simulink library "dsparch4"  (Simulink 8.0)
settings: Solver=ode45  SolverMode=SingleTasking  StartTime=0.0  StopTime=10.0  RelTol=1e-3
values from neighbouring files (symbols this model uses):
  a = ver('dsp')    [aboutdspsystbx.m]    (also in dsparch3Transform.m = localGetVal(inData.InstanceData, 'den', '1'); dspddes3Transform.m = sprintf('getYuleWalkerIIRFilterDesignOutput(; dspfdes.m = []; dsprprim.m = a-Mi)
  b = tmp(end-3:end)    [aboutdspsystbx.m]    (also in dsparch3Transform.m = localGetVal(inData.InstanceData, 'num', '[1 2]'); dspcsum.m = find_system(blk,'LookUnderMasks','all', 'FollowLinks','on', ; dspddes3Transform.m = sprintf('; dspfdes.m = [])
  c = []    [dspfdes.m]    (also in hdldspblks_control.m = hdlnewcontrol(mfilename); midicontrols.m = cell(1,midiCountDevices); midiid.m = onCleanup(@()cleanup(cids)))
  d = docroot    [dspbhelp.m]    (also in dspfdes.m = []; dsprprim.m = ['x[' num2str(Mi) 'n/' num2str(Li) ']'])
  D = D + B    [rebuffer_delay.m]
  H = reshape(H,Li,Mi*Ni)    [dsprprim.m]
  L = h.Length    [maxstep.m]    (also in msepred.m; msesim.m)
  M = 1    [msepred.m]    (also in msesim.m)
  N = str2double(s)    [dspcsum.m]    (also in dspddes3Transform.m = sprintf('; dspwdes.m = varargin{2}; if isempty(N), N=64; end)
undefined symbols (not defined in the file or in its folder): bitrevorder, dspblkfdatool
undefined symbols (not defined in the file): dfilt
libraries: dspmtrx3 x7, dspxfrm3 x4, dspsigattribs x3, dspsigops x2, dsparch4 x1
settings Model: FPTRunName=Active  Creator=hshivaku  LastModifiedBy=schim  ExtModeAutoUpdateStatusClock=off

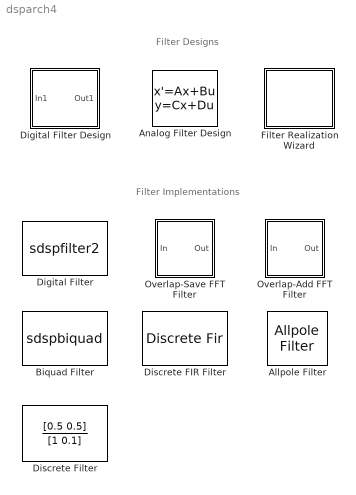
== system dsparch4 ==
  note: Filter Designs
  note: Filter Implementations
  Allpole Filter : AllpoleFilter
  Analog Filter Design : StateSpace  A=a  B=b  C=c  D=d  mask(Analog Filter Design){method=Butterworth, filttype=Lowpass, N=8, Wlo=30, Whi=80, Rp=2, Rs=40}
      mask prompts: method "Design method:"; filttype "Filter type:"; N "Filter order:"; Wlo "Passband edge frequency (rad/s):"; Whi "(unused)"; Rp "Passband ripple in dB:"; Rs "Stopband attenuation in dB:"
      mask help: Design one of several standard analog filters, implemented in state-space form.
      mask init:
      | [a,b,c,d,h,w,str]=dspblkanalog('design', method,filttype,N,Wlo,Whi,Rp,Rs);
      mask Help: eval('blocksethelp');
      mask TypeOptions method: Butterworth | Chebyshev I | Chebyshev II | Elliptic | Bessel
      mask Callback method: dspblkanalog
      mask TypeOptions filttype: Lowpass | Highpass | Bandpass | Bandstop
      mask Callback filttype: dspblkanalog
      mask Display: plot(w,h); text(.05,.9,str);
  Biquad Filter : S-Function  DialogController=dspdialog.BiquadFilter  DialogControllerArgs=DataTag1  FunctionName=sdspbiquad  Parameters=a.CoeffSource,a.FilterStruct,a.SOSCoeffs,a.ScaleValues,a.OptimizeScaleValues,a.ScaleValueMode,a.IC,a.ICnum,a.ICden,InputProcessing,dtInfo.arithmetic,dtInfo.inputWordLength,dtInfo.inputFracLength,dtInfo.secondCoeffFracLength,dtInfo.scaleValueFracLength,dtInfo.stageInputMode,dtInfo.stageOutputMode,dtInfo.stageInputWordLength,dtInfo.stageInputFracLength,dtInfo.stageOutputWordLength,dtInfo.stageOutputFracLength,dtInfo.multiplicandMode,dtInfo.multiplicandWordLength,dtInfo.multiplicandFracLength,dtInfo.denProdOutputFracLength, dtInfo.denAccumFracLength, dtInfo.denStateFracLength,dtInfo.firstCoeffMode,dtInfo.firstCoeffWordLength,dtInfo.firstCoeffFracLength,dtInfo.prodOutputMode,dtInfo.prodOutputWordLength,dtInfo.prodOutputFracLength,dtInfo.accumMode,dtInfo.accumWordLength,dtInfo.accumFracLength,dtInfo.memoryMode,dtInfo.memoryWordLength,dtInfo.memoryFracLength,dtInfo.outputMode,dtInfo.outputWordLength,dtInfo.outputFracLength,dtInfo.roundingMode,dtInfo.overflowMode  EnableBusSupport=off  mask(Biquad Filter){IIRFiltStruct=Direct form II transposed, CoeffSource=Specify via dialog, BiQuadCoeffs=[1 0.3 0.4 1 0.1 0.2], a0Flag=Warning, IC=0, ICnum=0, ICden=0, InputProcessing=Columns as channels (frame based), allowOverrides=on, firstCoeffMode=Same word length as input, firstCoeffWordLength=16, firstCoeffFracLength=15, secondCoeffMode=Same as numerator, secondCoeffWordLength=16, secondCoeffFracLength=15, outputMode=Same as accumulator, outputWordLength=16, outputFracLength=15, accumMode=Same as product output, accumWordLength=32, accumFracLength=30, denAccumFracLength=30, prodOutputMode=Same as input, prodOutputWordLength=32, prodOutputFracLength=30, denProdOutputFracLength=30, memoryMode=Same as accumulator, memoryWordLength=16, memoryFracLength=15, secondMemoryFracLength=15, roundingMode=Floor, overflowMode=off, ScaleValues=1, optimizeScaleValues=on, ScaleValueMode=Specify via input port (g), scaleValueFracLength=14, stageInputMode=Same as input, stageOutputMode=Same as section input, stageInputWordLength=16, stageInputFracLength=15, stageOutputWordLength=16, stageOutputFracLength=15, LockScale=off, FilterSource=Specify via dialog, dfiltObjectName=dfilt.df2tsos([1 0.3 0.4],[1 0.1 0.2]), multiplicandMode=Same as output, multiplicandWordLength=32, multiplicandFracLength=30}
      mask prompts: IIRFiltStruct "Filter structure:"; CoeffSource "Coefficient source:"; BiQuadCoeffs "SOS matrix (Mx6):"; a0Flag "Action when the values on the fourth column of the SOS matrix (a01...a0M) are not one:"; IC "Initial conditions:"; ICnum "Initial conditions on zeros side:"; ICden "Initial conditions on poles side:"; InputProcessing "Input processing:"; allowOverrides "Allow overrides from DSP Fixed-Point Attributes blocks"; firstCoeffMode "Numerator coefficient attributes:"; firstCoeffWordLength "Numerator coefficient word length:"; firstCoeffFracLength "Numerator coefficient fraction length:"; secondCoeffMode "Denominator coefficient attributes:"; secondCoeffWordLength "Denominator coefficient word length:"; secondCoeffFracLength "Denominator coefficient fraction length:"; outputMode "Output attributes:"; outputWordLength "Output word length:"; outputFracLength "Output fraction length:"; accumMode "Accumulator attributes:"; accumWordLength "Accumulator word length:"; accumFracLength "Accumulator fraction length:"; denAccumFracLength "Den accumulator fraction length:"; prodOutputMode "Product output attributes:"; prodOutputWordLength "Product output word length:"; prodOutputFracLength "Product output fraction length:"; denProdOutputFracLength "Den product output fraction length:"; memoryMode "State memory attributes:"; memoryWordLength "State memory word length:"; memoryFracLength "State memory fraction length:"; secondMemoryFracLength "Den state memory fraction length:"; roundingMode "Round integer calculations toward:"; overflowMode "Saturate on integer overflow"; ScaleValues "Scale values:"; optimizeScaleValues "Replace unity scale values with a signal line:"; ScaleValueMode "Scale values mode:"; scaleValueFracLength "Scale value fraction length:"; stageInputMode "Stage Input attributes:"; stageOutputMode "Stage output attributes:"; stageInputWordLength "Stage input word length:"; stageInputFracLength "Stage input fraction length:"; stageOutputWordLength "Stage output word length:"; stageOutputFracLength "State output fraction length:"; LockScale "Lock scaling"; FilterSource "Filter source:"; dfiltObjectName "Discrete-time filter variable:"; multiplicandMode "Multiplicand attributes:"; multiplicandWordLength "Multiplicand word length:"; multiplicandFracLength "Multiplicand fraction length:"
      mask help: Implement a general IIR filter using biquad structures. Biquad implementations of general IIR filters are often preferred due to their desirable numeric properties.
      mask init:
      | s           = dspblkbiquad3('icon');
      | [a, dtInfo] = dspblkbiquad3('getDefaults');
      | if FilterSource == 3
      |    [a, dtInfo] = dspblkbiquad3('init',dfiltObjectName);
      | else
      |     paramValues.BiQuadCoeffs = BiQuadCoeffs;
      |     paramValues.ScaleValues = ScaleValues;
      |     paramValues.OptimizeScaleValues = optimizeScaleValues;
      |     paramValues.ScaleValueMode = ScaleValueMode;
      |     paramValues.IC = IC;
      |     paramValues.ICnum = ICnum;
      |     paramValues.ICden = ICden;
      |     paramValues.a0Flag = a0Flag;
      |     [a, dtInfo] = dspblkbiquad3('init',paramValues);
      | end
      settings: DeleteFcn=dspLinkFVTool2Mask(gcbh,'close')  ModelCloseFcn=dspLinkFVTool2Mask(gcbh,'close')  CloseFcn=dspLinkFVTool2Mask(gcbh,'close')
      mask Help: eval('blocksethelp');
      mask TypeOptions IIRFiltStruct: Direct form I | Direct form I transposed | Direct form II | Direct form II transposed
      mask TypeOptions CoeffSource: Specify via dialog | Input port(s) | dfilt object
      mask TypeOptions a0Flag: None | Warning | Error
      mask TypeOptions InputProcessing: Columns as channels (frame based) | Elements as channels (sample based) | Inherited (this choice will be removed - see release notes)
      mask TypeOptions firstCoeffMode: Same word length as input | Specify word length | Binary point scaling | Slope and bias scaling | Same as input | User-defined
      mask TypeOptions secondCoeffMode: Same as numerator | Same word length as numerator | Same word length as input | Binary point scaling | Slope and bias scaling | Same as input | User-defined
      mask TypeOptions outputMode: Same as input | Same as accumulator | Binary point scaling | Slope and bias scaling | User-defined
      mask TypeOptions accumMode: Same as input | Same as product output | Binary point scaling | Slope and bias scaling | User-defined
      mask TypeOptions prodOutputMode: Same as input | Binary point scaling | Slope and bias scaling | User-defined
      mask TypeOptions memoryMode: Same as input | Same as accumulator | Binary point scaling | Slope and bias scaling | User-defined
      mask TypeOptions roundingMode: Ceiling | Convergent | Floor | Nearest | Round | Simplest | Zero
      mask TypeOptions ScaleValueMode: Specify via input port (g) | Assume all are unity and optimize
      mask TypeOptions stageInputMode: Same as input | Binary point scaling | Slope and bias scaling
      mask TypeOptions stageOutputMode: Same as section input | Binary point scaling | Slope and bias scaling
      mask TypeOptions FilterSource: Specify via dialog | Input port(s) | dfilt object
      mask TypeOptions multiplicandMode: Same as output | Binary point scaling | Slope and bias scaling
      mask Display:
      | text(s.posx,s.posy,s.icon,'horiz','center');
      | port_label('input',s.i1,s.s1);
      | port_label('input',s.i2,s.s2);
      | port_label('input',s.i3,s.s3);
      | port_label('input',1,s.in);
      | port_label('output',1,s.out);
  Digital Filter Design : Subsystem  StartFcn=dspblkfdatool('StartFcn');  mask(Digital Filter Design){mwdsp_browser_bugfix_var=off}
      mask prompts: mwdsp_browser_bugfix_var "Dummy variable to fix library browser display bug"
      mask help: Launches FDATool to design and implement single-rate filters using the Digital Filter block.
      mask init:
      | [h, err] = dspblkfdatool('initializationCommands');
      | if ~isempty(err)
      |     rethrow(err);
      | end
      settings: ModelCloseFcn=dspblkfdatool('ModelCloseFcn');  NameChangeFcn=dspblkfdatool('NameChange');  OpenFcn=dspblkfdatool('OpenFcn');  CloseFcn=dspblkfdatool('CloseFcn');
      mask Help: eval('blocksethelp');
      mask Display:
      | plot(h);
      | text(.05,.9,'FDATool')
  Digital Filter : S-Function  DialogController=dspdialog.DigitalFilter  DialogControllerArgs=DataTag5  FunctionName=sdspfilter2  Parameters=a.CoeffSource,a.FilterType,a.FilterStruct,a.FilterPerSample,a.a0CoeffIsUnity,NumCoeffs,DenCoeffs,LatticeCoeffs,a.SOSCoeffs,a.ScaleValues,a.IC,a.ICnum,a.ICden,InputProcessing,dtInfo.arithmetic,dtInfo.inputWordLength,dtInfo.inputFracLength,dtInfo.secondCoeffFracLength,dtInfo.scaleValueFracLength,dtInfo.tapSumMode,dtInfo.tapSumWordLength,dtInfo.tapSumFracLength,dtInfo.sectionIOMode,dtInfo.sectionIOWordLength,dtInfo.sectionInWordLength,dtInfo.sectionInFracLength,dtInfo.sectionOutWordLength,dtInfo.sectionOutFracLength,dtInfo.multiplicandMode,dtInfo.multiplicandWordLength,dtInfo.multiplicandFracLength,dtInfo.denProdOutputFracLength,dtInfo.denAccumFracLength,dtInfo.denStateFracLength,dtInfo.firstCoeffMode,dtInfo.firstCoeffWordLength,dtInfo.firstCoeffFracLength,dtInfo.prodOutputMode,dtInfo.prodOutputWordLength,dtInfo.prodOutputFracLength,dtInfo.accumMode,dtInfo.accumWordLength,dtInfo.accumFracLength,dtInfo.memoryMode,dtInfo.memoryWordLength,dtInfo.memoryFracLength,dtInfo.outputMode,dtInfo.outputWordLength,dtInfo.outputFracLength,dtInfo.roundingMode,dtInfo.overflowMode  EnableBusSupport=off  mask(Digital Filter){TypePopup=IIR (poles & zeros), IIRFiltStruct=Direct form II transposed, AllPoleFiltStruct=Direct form, FIRFiltStruct=Direct form, CoeffSource=Specify via dialog, NumCoeffs=[1 2], DenCoeffs=[1 0.1], BiQuadCoeffs=[1 0.3 0.4 1 0.1 0.2], LatticeCoeffs=[0.2 0.4], denIgnore=on, FiltPerSampPopup=One filter per frame, IC=0, ICnum=0, ICden=0, additionalParams=off, allowOverrides=on, showCoeff=off, firstCoeffMode=Same word length as input, firstCoeffWordLength=16, firstCoeffFracLength=15, secondCoeffMode=Same as numerator, secondCoeffWordLength=16, secondCoeffFracLength=15, thirdCoeffMode=Same as input, thirdCoeffWordLength=16, thirdCoeffFracLength=15, showOut=off, outputMode=Same as accumulator, outputWordLength=16, outputFracLength=15, showAcc=off, accumMode=Same as product output, accumWordLength=32, accumFracLength=30, showMpy=off, prodOutputMode=Same as input, prodOutputWordLength=32, prodOutputFracLength=30, showMem=off, memoryMode=Same as accumulator, memoryWordLength=16, memoryFracLength=15, roundingMode=Floor, overflowMode=off, ScaleValues=1, scaleValueFracLength=14, tapSumMode=Same as input, tapSumWordLength=32, tapSumFracLength=30, stageIOMode=Same as input, stageIOWordLength=16, stageInFracLength=15, stageOutFracLength=15, LockScale=off, FilterSource=Specify via dialog, dfiltObjectName=dfilt.dffir([1 2 1]), multiplicandMode=Same as output, multiplicandWordLength=32, multiplicandFracLength=30, InputProcessing=Columns as channels (frame based)}
      mask prompts: TypePopup "Transfer function type:"; IIRFiltStruct "Filter structure:"; AllPoleFiltStruct "Filter structure:"; FIRFiltStruct "Filter structure:"; CoeffSource "Coefficient source:"; NumCoeffs "Numerator coefficients:"; DenCoeffs "Denominator coefficients:"; BiQuadCoeffs "SOS matrix (Mx6):"; LatticeCoeffs "Reflection coefficients:"; denIgnore "First denominator coefficient = 1, remove 1/a0 term in the structure"; FiltPerSampPopup "Coefficient update rate:"; IC "Initial conditions:"; ICnum "Initial conditions on zeros side:"; ICden "Initial conditions on poles side:"; additionalParams "------- Show additional parameters --------"; allowOverrides "Allow overrides from DSP Fixed-Point Attributes blocks"; showCoeff "------- Show coefficient fixed-point attributes --------"; firstCoeffMode "Numerator coefficient attributes:"; firstCoeffWordLength "Numerator coefficient word length:"; firstCoeffFracLength "Numerator coefficient fraction length:"; secondCoeffMode "Denominator coefficient attributes:"; secondCoeffWordLength "Denominator coefficient word length:"; secondCoeffFracLength "Denominator coefficient fraction length:"; thirdCoeffMode "Denominator coefficient attributes:"; thirdCoeffWordLength "Denominator coefficient word length:"; thirdCoeffFracLength "Denominator coefficient fraction length:"; showOut "------- Show output fixed-point attributes --------"; outputMode "Output attributes:"; outputWordLength "Output word length:"; outputFracLength "Output fraction length:"; showAcc "------- Show accumulator fixed-point attributes --------"; accumMode "Accumulator attributes:"; accumWordLength "Accumulator word length:"; accumFracLength "Accumulator fraction length:"; showMpy "------- Show product output fixed-point attributes --------"; prodOutputMode "Product output attributes:"; prodOutputWordLength "Product output word length:"; prodOutputFracLength "Product output fraction length:"; showMem "------- Show state memory fixed-point attributes --------"; memoryMode "State memory attributes:"; memoryWordLength "State memory word length:"; memoryFracLength "State memory fraction length:"; roundingMode "Round integer calculations toward:"; overflowMode "Saturate on integer overflow"; ScaleValues "Scale values:"; scaleValueFracLength "Scale value fraction length:"; tapSumMode "Tap sum attributes:"; tapSumWordLength "Tap sum word length:"; tapSumFracLength "Tap sum fraction length:"; stageIOMode "Stage IO attributes:"; stageIOWordLength "Stage IO word length:"; stageInFracLength "Stage input fraction length:"; stageOutFracLength "Stage output fraction length:"; LockScale "Lock scaling"; FilterSource "Filter source:"; dfiltObjectName "Discrete-time filter variable:"; multiplicandMode "Multiplicand attributes:"; multiplicandWordLength "Multiplicand word length:"; multiplicandFracLength "Multiplicand fraction length:"; InputProcessing "Input processing:"
      mask help: Independently filter each channel of the input over time using a specified digital filter implementation. You can specify filter coefficients using either tunable mask dialog parameters or separate input ports, which are useful for time-varying coefficients.
      mask init:
      | s           = dspblkfilter('icon');
      | [a, dtInfo] = dspblkfilter('getDefaults');
      | if FilterSource == 3
      |     [a, dtInfo] = dspblkfilter('init',dfiltObjectName);
      |     NumCoeffs = a.NumCoeffs;
      |     DenCoeffs = a.DenCoeffs;
      |     LatticeCoeffs = a.LatticeCoeffs;
      | else
      |     paramValues.NumCoeffs = NumCoeffs;
      |     paramValues.DenCoeffs = DenCoeffs;
      |     paramValues.LatticeCoeffs = LatticeCoeffs;
      |     paramValues.BiQuadCoeffs = BiQuadCoeffs;
      |     paramValues.ScaleValues = ScaleValues;
      |     paramValues.IC = IC;
      |     paramValues.ICnum = ICnum;
      |     paramValues.ICden = ICden;
      |     [a, dtInfo] = dspblkfilter('init',paramValues);
      | end
      settings: DeleteFcn=dspLinkFVTool2Mask(gcbh,'close')  ModelCloseFcn=dspLinkFVTool2Mask(gcbh,'close')  CloseFcn=dspLinkFVTool2Mask(gcbh,'close')
      mask Help: eval('blocksethelp');
      mask TypeOptions TypePopup: IIR (poles & zeros) | IIR (all poles) | FIR (all zeros)
      mask Callback TypePopup: dspblkfilter('dynamic');
      mask TypeOptions IIRFiltStruct: Direct form I | Direct form I transposed | Direct form II | Direct form II transposed | Biquad direct form I (SOS) | Biquad direct form I transposed (SOS) | Biquad direct form II (SOS) | Biquad direct form II transposed (SOS)
      mask TypeOptions AllPoleFiltStruct: Direct form | Direct form transposed | Lattice AR
      mask TypeOptions FIRFiltStruct: Direct form | Direct form symmetric | Direct form antisymmetric | Direct form transposed | Lattice MA
      mask TypeOptions CoeffSource: Specify via dialog | Input port(s)
      mask TypeOptions FiltPerSampPopup: One filter per frame | One filter per sample
      mask TypeOptions firstCoeffMode: Same word length as input | Specify word length | Binary point scaling | Slope and bias scaling | Same as input | User-defined
      mask TypeOptions secondCoeffMode: Same as numerator | Same word length as numerator | Same word length as input | Binary point scaling | Slope and bias scaling | Same as input | User-defined
      mask TypeOptions thirdCoeffMode: Same word length as input | Binary point scaling | Slope and bias scaling | Same as input | User-defined
      mask TypeOptions outputMode: Same as input | Same as accumulator | Binary point scaling | Slope and bias scaling | User-defined
      mask TypeOptions accumMode: Same as input | Same as product output | Binary point scaling | Slope and bias scaling | User-defined
      mask TypeOptions prodOutputMode: Same as input | Binary point scaling | Slope and bias scaling | User-defined
      mask TypeOptions memoryMode: Same as input | Same as accumulator | Binary point scaling | Slope and bias scaling | User-defined
      mask TypeOptions roundingMode: Ceiling | Convergent | Floor | Nearest | Round | Simplest | Zero
      mask TypeOptions tapSumMode: Same as input | Binary point scaling | Slope and bias scaling
      mask TypeOptions stageIOMode: Same as input | Binary point scaling | Slope and bias scaling
      mask TypeOptions FilterSource: Specify via dialog | Input port(s) | dfilt object
      mask TypeOptions multiplicandMode: Same as output | Binary point scaling | Slope and bias scaling
      mask TypeOptions InputProcessing: Columns as channels (frame based) | Elements as channels (sample based) | Inherited (this choice will be removed - see release notes)
      mask Display:
      | text(s.posx,s.posy,s.icon,'horiz','center');
      | port_label('input',s.i1,s.s1);
      | port_label('input',s.i2,s.s2);
      | port_label('input',1,s.in);
      | port_label('output',1,s.out);
  Discrete FIR Filter : DiscreteFir  InputProcessing=Columns as channels (frame based)
  Discrete Filter : DiscreteFilter  Numerator=[0.5 0.5]  Denominator=[1 0.1]  InputProcessing=Columns as channels (frame based)  FilterStructure=Direct form II transposed  a0EqualsOne=on
  Filter Realization Wizard : Subsystem  mask(Filter Realization Wizard){}
      mask help: Automatically construct filter realizations with specific architectures, using sum, gain, and delay blocks.
      mask init:
      | xw=[NaN 0.8 0.8 NaN 0.687 0.743 NaN 0.64 0.72 NaN 0.710 0.743 NaN 0.8 0.8 NaN 0.913 0.857 NaN 0.96 0.88 NaN 0.808 0.792 0.961 0.978 0.808 NaN 0.825 0.808 NaN 0.961 0.944];
      | yw=[NaN 0.64 0.72 NaN 0.687 0.743 NaN 0.8 0.8 NaN 0.890 0.857 NaN 0.96 0.88 NaN 0.913 0.857 NaN 0.8 0.8 NaN 0.808 0.792 0.622 0.639 0.808 NaN 0.792 0.775 NaN 0.656 0.639];
      | 
      | xl = [.1 .7 NaN .3 .3 NaN .7 .7 NaN .3 .3 NaN .7 .7 NaN .3 .9];
      | yl = [.8 .8 NaN .8 .6 NaN .8 .6 NaN .4 .2 NaN .4 .13 NaN .2 .2];
      | xz = [.46 .54 .46 NaN .54 .59 .54 .59 NaN .61 .64 NaN .67 .67];
      | yz = [.84 .8  .76 NaN .92 .92 .86 .86 NaN .93 .93 NaN .97 .89];
      | xg = [.21 .39 .3 .21 NaN .61 .79 .7 .61];
      | yg = [.6  .6  .4 .6  NaN .6  .6  .4 .6];
      | t=(0:12)/12*2*pi;
      | xs = .07*cos(t)+.7;
      | ys = .07*sin(t)+.2;
      settings: OpenFcn=dspfwiz
      mask Help: eval('blocksethelp');
      mask Display:
      | text(.05, .9, 'FDATool');
      | plot([[xl NaN xz NaN xg NaN xs NaN]*.9-.075 xw],[[yl NaN yz NaN yg NaN ys NaN]*.9-.1 yw]);
  Overlap-Add FFT Filter : Subsystem  mask(Overlap-Add FFT Filter){Nfft=64, h=fir1(20,0.2), output_complexity=Real, TreatMby1Signals=One channel}
      mask prompts: Nfft "FFT size:"; h "FIR coefficients:"; output_complexity "Output:"; TreatMby1Signals "Treat Mx1 and unoriented sample-based signals as:"
      mask help:
      | FFT based filtering using the overlap-add algorithm. Set 'Output' to 'Complex' if either the input signal or the filter coefficients are complex.
      |
      | 'FFT Size' must equal or exceed the number of filter coefficients.  Smaller FFT sizes lead to less latency but also less computational efficiency, decreasing the benefits of frequency domain processing.
      mask init:
      | [N,H,M,L] = dspblkolapfilt(gcb,'init',double(Nfft),h,'Overlap-Add');
      mask Help: eval('blocksethelp');
      mask TypeOptions output_complexity: Real | Complex
      mask TypeOptions TreatMby1Signals: One channel | M channels (this choice will be removed - see release notes)
      mask Display:
      | disp('Overlap\nAdd');
      | ... plot(log10(abs(H(1:(N/2)))))
  Overlap-Save FFT Filter : Subsystem  mask(Overlap-Save FFT Filter){nfft_in=64, h=fir1(20,0.2), output_complexity=Real, TreatMby1Signals=One channel}
      mask prompts: nfft_in "FFT size:"; h "FIR coefficients:"; output_complexity "Output:"; TreatMby1Signals "Treat Mx1 and unoriented sample-based signals as:"
      mask help:
      | FFT based filtering using the overlap-save algorithm.  Set 'Output' to 'Complex' if either the input signal or the filter coefficients are complex.
      |
      | 'FFT Size' must equal or exceed the number of filter coefficients.  Smaller FFT sizes lead to less latency but also less computational efficiency, decreasing the benefits of frequency domain processing.
      mask init:
      | [N,H,M] = dspblkolapfilt(gcb,'init',double(nfft_in),h,'Overlap-Save');
      mask Help: eval('blocksethelp');
      mask TypeOptions output_complexity: Real | Complex
      mask TypeOptions TreatMby1Signals: One channel | M channels (this choice will be removed - see release notes)
      mask Display:
      | disp('Overlap\nSave');
      | ... plot(log10(abs(H(1:(nfft/2)))))

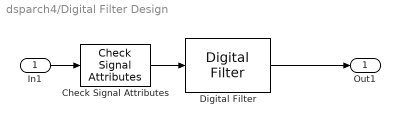
== system dsparch4/Digital Filter Design ==
  In1 : Inport
  Check Signal Attributes : dspsigattribs/Check Signal Attributes  SystemSampleTime=-1  SigAttribCheckMethod=Does not match attributes exactly  Complexity=Ignore  Frame=Ignore  DimsCheckMethod=Ignore  Dimensions=1-D  DatatypeCheckMethod=Is...  DatatypeGeneral=Floating-point  DtypeFloatSpecific=Any floating-point  DtypeFixedSpecific=Any fixed-point  DtypeIntSpecific=Any integer  SampleMode=Ignore
  Digital Filter : dsparch4/Digital Filter  TypePopup=FIR (all zeros)  IIRFiltStruct=Direct form II transposed  AllPoleFiltStruct=Direct form  FIRFiltStruct=Direct form  CoeffSource=Specify via dialog  NumCoeffs=[-0.000922175232821972001 -0.00273958133317832222 -0.00255036555988357068 0.00355621457714135319 0.0135493675450093672 0.01731581678436514 0.00770838306531652657 -0.00649307059052154061 -0.00768045146622221581 0.00608565944583592047 0.0138781398261133507 0.000396827974269109223 -0.0168728258912879542 -0.00891939395727656126 0.0174119503029707412 0.0207545927500638709 -0.0122604496044704976 -0.0342350688782289414 -0.0010657411785084522 0.0477779205992945599 0.0273960894331456359 -0.0593497624727358716 -0.0823259890492310659 0.067152220451342684 0.310023479333045027 0.43008758517821305 0.310023479333045027 0.067152220451342684 -0.0823259890492310659 -0.0593497624727358716 0.0273960894331456359 0.0477779205992945599 -0.0010657411785084522 -0.0342350688782289414 -0.0122604496044704976 0.0207545927500638709 0.0174119503029707412 -0.00891939395727656126 -0.0168728258912879542 0.000396827974269109223 0.0138781398261133507 0.00608565944583592047 -0.00768045146622221581 -0.00649307059052154061 0.00770838306531652657 0.01731581678436514 0.0135493675450093672 0.00355621457714135319 -0.00255036555988357068 -0.00273958133317832222 -0.000922175232821972001]  DenCoeffs=[1 0.1]  BiQuadCoeffs=[1 0.3 0.4 1 0.1 0.2]  LatticeCoeffs=[0.2 0.4]  denIgnore=on  FiltPerSampPopup=One filter per frame  IC=0  ICnum=0  ICden=0  roundingMode=Floor  overflowMode=off  ScaleValues=1  scaleValueFracLength=14  stageInFracLength=15  stageOutFracLength=15  FilterSource=Specify via dialog  dfiltObjectName=0  InputProcessing=Columns as channels (frame based)
  Out1 : Outport
  wires:
  In1/1 -> Check Signal Attributes/1
  Digital Filter/1 -> Out1/1
  Check Signal Attributes/1 -> Digital Filter/1

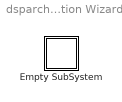
== system dsparch4/Filter Realization Wizard ==
  Empty SubSystem : Subsystem

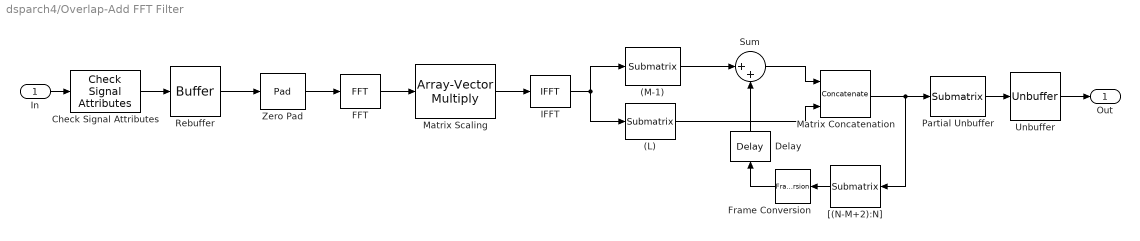
== system dsparch4/Overlap-Add FFT Filter ==
  In : Inport
  (L) : dspmtrx3/Submatrix  RowSpan=Range of rows  RowStartMode=Offset from last  RowStartIndex=L-1  RowEndMode=Last  RowEndIndex=1  ColSpan=All columns  ColStartMode=First  ColStartIndex=1  ColEndMode=Last  ColEndIndex=1
  (M-1) : dspmtrx3/Submatrix  RowSpan=Range of rows  RowStartMode=First  RowStartIndex=M-1  RowEndMode=Index  RowEndIndex=M-1  ColSpan=All columns  ColStartMode=First  ColStartIndex=1  ColEndMode=Last  ColEndIndex=1
  Check Signal Attributes : dspsigattribs/Check Signal Attributes  SystemSampleTime=-1  SigAttribCheckMethod=Does not match attributes exactly  Complexity=Ignore  Frame=Ignore  DimsCheckMethod=Ignore  Dimensions=1-D  DatatypeCheckMethod=Is...  DatatypeGeneral=Floating-point  DtypeFloatSpecific=Any floating-point  DtypeFixedSpecific=Any fixed-point  DtypeIntSpecific=Any integer  SampleMode=Ignore
  Delay : dspsigops/Delay  dly_unit=Samples  delay=1  ic_detail=off  dif_ic_for_ch=off  dif_ic_for_dly=off  ic=0  reset_popup=None
  FFT : dspxfrm3/FFT  CompMethod=Table lookup  TableOpt=HYBRID  TableOptActive=Speed  BitRevOrder=on  InheritFFTLength=on  FFTLength=64  RowConvenienceOn=on  FFTImplementation=Auto  SkipNorm=off  firstCoeffDataTypeStr=Inherit: Same word length as input  firstCoeffLastDataTypeStr=Inherit: Same word length as input  outputMin=[]  outputMax=[]  roundingMode=Floor  overflowMode=off
      settings: allowOverrides=off
  Frame Conversion : FrameConversion  OutFrame=Sample-based
  IFFT : dspxfrm3/IFFT  CompMethod=Table lookup  TableOpt=HYBRID  TableOptActive=Speed  BitRevOrder=on  cs_in=on  SkipNorm=on  InheritFFTLength=on  FFTLength=64  mode=Real  outSamplingMode=Frame based  RowConvenienceOn=on  FFTImplementation=Auto  firstCoeffDataTypeStr=Inherit: Same word length as input  firstCoeffLastDataTypeStr=Inherit: Same word length as input  outputMin=[]  outputMax=[]  roundingMode=Floor  overflowMode=off
      settings: allowOverrides=off
  Matrix Concatenation : Concatenate  Mode=Multidimensional array
  Matrix Scaling : dspmtrx3/Array-Vector Multiply  mode=Mute  saveAsFlag=0  Dimension=1  V_Source=Dialog parameter  V_VectFromMask=bitrevorder(H(:))  firstCoeffSignedness=Auto  firstCoeffDataTypeStr=Inherit: Same word length as input  firstCoeffLastDataTypeStr=Inherit: Same word length as input  firstCoeffMin=[]  firstCoeffMax=[]  outputSignedness=Auto  outputDataTypeStr=Inherit: Same as product output  outputLastDataTypeStr=Inherit: Same as product output  outputMin=[]  outputMax=[]  accumSignedness=Auto  prodOutputSignedness=Auto  roundingMode=Floor  overflowMode=off
      settings: allowOverrides=off
  Partial Unbuffer : dspmtrx3/Submatrix  RowSpan=Range of rows  RowStartMode=First  RowStartIndex=M  RowEndMode=Index  RowEndIndex=L  ColSpan=All columns  ColStartMode=First  ColStartIndex=1  ColEndMode=Last  ColEndIndex=1
  Rebuffer : Buffer  N=44  TreatMby1Signals=One channel
  Sum : Sum  Inputs=|++  InputSameDT=on
  Unbuffer : Unbuffer  SampleBasedProcessing=Same as frame based
  Zero Pad : dspsigops/Pad  padAlong=Columns  dimsToPad=1  valSrc=Specify via dialog  padVal=0  spec=Output size  padNumOutRowsSpecMethod=User-specified  numOutRows=N  padNumOutColsSpecMethod=User-specified  numOutCols=1  isVarDimsMode=off  padBeginning=0  padEnd=0  outSizeMode=User-specified  outSize=1  padSigAt=End  trunc_flag=None  roundingMode=Floor  overflowMode=off  truncOrWrapMode=Truncate  wrap_flag=None
  "[(N-M+2):N]" : dspmtrx3/Submatrix  RowSpan=Range of rows  RowStartMode=Index  RowStartIndex=(N-M+2)  RowEndMode=Last  RowEndIndex=N  ColSpan=All columns  ColStartMode=First  ColStartIndex=1  ColEndMode=Last  ColEndIndex=1
  Out : Outport  InitialOutput=0
  wires:
  Partial Unbuffer/1 -> Unbuffer/1
  Sum/1 -> Matrix Concatenation/1
  (M-1)/1 -> Sum/1
  Delay/1 -> Sum/2
  (L)/1 -> Matrix Concatenation/2
  "[(N-M+2):N]"/1 -> Frame Conversion/1
  Matrix Concatenation/1 -> Partial Unbuffer/1, "[(N-M+2):N]"/1
  Unbuffer/1 -> Out/1
  Matrix Scaling/1 -> IFFT/1
  IFFT/1 -> (L)/1, (M-1)/1
  Zero Pad/1 -> FFT/1
  Rebuffer/1 -> Zero Pad/1
  FFT/1 -> Matrix Scaling/1
  In/1 -> Check Signal Attributes/1
  Frame Conversion/1 -> Delay/1
  Check Signal Attributes/1 -> Rebuffer/1

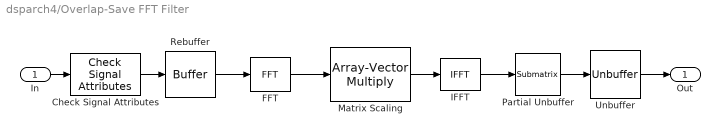
== system dsparch4/Overlap-Save FFT Filter ==
  In : Inport
  Check Signal Attributes : dspsigattribs/Check Signal Attributes  SystemSampleTime=-1  SigAttribCheckMethod=Does not match attributes exactly  Complexity=Ignore  Frame=Ignore  DimsCheckMethod=Ignore  Dimensions=1-D  DatatypeCheckMethod=Is...  DatatypeGeneral=Floating-point  DtypeFloatSpecific=Any floating-point  DtypeFixedSpecific=Any fixed-point  DtypeIntSpecific=Any integer  SampleMode=Ignore
  FFT : dspxfrm3/FFT  CompMethod=Table lookup  TableOpt=HYBRID  TableOptActive=Speed  BitRevOrder=on  InheritFFTLength=on  FFTLength=64  RowConvenienceOn=on  FFTImplementation=Auto  SkipNorm=off  firstCoeffDataTypeStr=Inherit: Same word length as input  firstCoeffLastDataTypeStr=Inherit: Same word length as input  outputMin=[]  outputMax=[]  roundingMode=Floor  overflowMode=off
      settings: allowOverrides=off
  IFFT : dspxfrm3/IFFT  CompMethod=Table lookup  TableOpt=HYBRID  TableOptActive=Speed  BitRevOrder=on  cs_in=on  SkipNorm=on  InheritFFTLength=on  FFTLength=64  mode=Real  outSamplingMode=Frame based  RowConvenienceOn=on  FFTImplementation=Auto  firstCoeffDataTypeStr=Inherit: Same word length as input  firstCoeffLastDataTypeStr=Inherit: Same word length as input  outputMin=[]  outputMax=[]  roundingMode=Floor  overflowMode=off
      settings: allowOverrides=off
  Matrix Scaling : dspmtrx3/Array-Vector Multiply  mode=Mute  saveAsFlag=0  Dimension=1  V_Source=Dialog parameter  V_VectFromMask=bitrevorder(H(:))  firstCoeffSignedness=Auto  firstCoeffDataTypeStr=Inherit: Same word length as input  firstCoeffLastDataTypeStr=Inherit: Same word length as input  firstCoeffMin=[]  firstCoeffMax=[]  outputSignedness=Auto  outputDataTypeStr=Inherit: Same as product output  outputLastDataTypeStr=Inherit: Same as product output  outputMin=[]  outputMax=[]  accumSignedness=Auto  prodOutputSignedness=Auto  roundingMode=Floor  overflowMode=off
      settings: allowOverrides=off
  Partial Unbuffer : dspmtrx3/Submatrix  RowSpan=Range of rows  RowStartMode=Index  RowStartIndex=M  RowEndMode=Last  RowEndIndex=1  ColSpan=All columns  ColStartMode=First  ColStartIndex=1  ColEndMode=Last  ColEndIndex=1
  Rebuffer : Buffer  V=20  TreatMby1Signals=One channel
  Unbuffer : Unbuffer  SampleBasedProcessing=Same as frame based
  Out : Outport  InitialOutput=0
  wires:
  Unbuffer/1 -> Out/1
  Partial Unbuffer/1 -> Unbuffer/1
  IFFT/1 -> Partial Unbuffer/1
  Matrix Scaling/1 -> IFFT/1
  Rebuffer/1 -> FFT/1
  FFT/1 -> Matrix Scaling/1
  In/1 -> Check Signal Attributes/1
  Check Signal Attributes/1 -> Rebuffer/1

== system dsparch4/Filter Realization Wizard/Empty SubSystem ==
